simulink subsystem "StreetLaneSegment1x2_asSubsystem"  (R2021a)
settings: Solver=VariableStepAuto  StartTime=0.0  StopTime=10.0  RelTol=1e-3
settings Model: Creator=phill  LastModifiedBy=phill

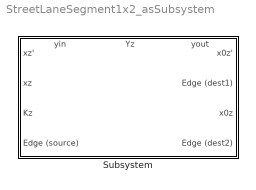
== system StreetLaneSegment1x2_asSubsystem ==
  Subsystem : Subsystem  mask{Kz=0, Tz=0}
      mask prompts: Kz "Kz (Capacity - How many cars fit into this cell)"; Tz "Tz (Nominal travel time for vehicles traveling unobstructed through the cell)"
      mask help: 1x2 Version of the 1x1 default cell.
      settings: PortSchema="{\"entries\":[{\"content\":{\"sides\":[{\"content\":{\"connectorIds\":[\"Out6\",\"Out7\",\"Out8\",\"In1\"]},\"type\":\"ConnectorPlacement.EquallySpacedRectSide\",\"uuid\":\"c6485919-43c0-4a3b-9a67-3a50a1748552\"},{\"content\":{\"connectorIds\":[\"Out1\",\"In2\",\"Out2\",\"In3\"],\"side\":\"RIGHT\"},\"type\":\"ConnectorPlacement.EquallySpacedRectSide\",\"uuid\":\"e12fc750-a76b-4a52-a085-56205ebef983\"},{\"content\":{\"connectorIds\":[\"Out3\",\"Out4\",\"Out5\"],\"side\":\"TOP\"},\"type\":\"ConnectorPlacement.EquallySpacedRectSide\",\"uuid\":\"04ec9430-4292-4c0e-9b60-ad78ee5b6ee3\"}]},\"type\":\"ConnectorPlacement.EquallySpacedConnector\",\"uuid\":\"8d657383-4de4-4f3e-906b-2968264a5f3c\"}],\"packageUris\":[\"http://schema.mathworks.com/mf0/Connector/R2020b\"],\"version\":\"1.0\"}"
      mask Display:
      | image('$imagefile'); % Use "Edit Image" on toolstrip to change.
      | %image('.\LaneIconLightGrey.png');
      | disp('Street Lane Segment 1x2 \n\n');
      | disp(['Kz = ', get_param(gcb,'Kz'), ' | Tz = ', get_param(gcb, 'Tz')])

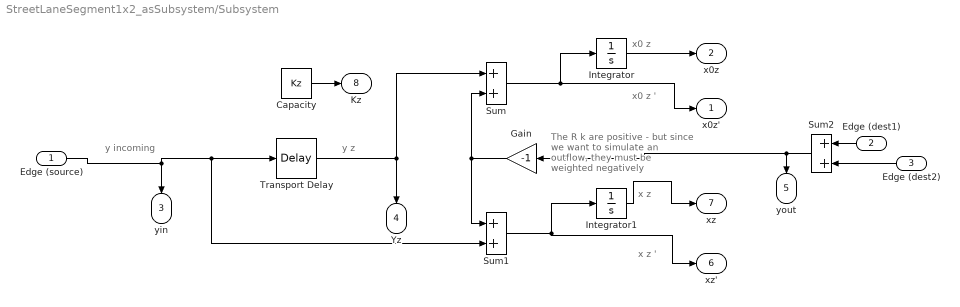
== system StreetLaneSegment1x2_asSubsystem/Subsystem ==
  note: The R k are positive - but since we
      | want to simulate an outflow, they
      | must be weighted negatively
  note: x0 z '
  note: y incoming
  note: y z
  note: x z
  note: x0 z
  note: x z '
  Edge (source) : Inport
  Edge (dest1) : Inport  Port=2
  Edge (dest2) : Inport  Port=3
  Capacity : Constant  Value=Kz
  Gain : Gain  Gain=-1
  Integrator : Integrator
  Integrator1 : Integrator
  Sum : Sum
  Sum1 : Sum
  Sum2 : Sum
  Transport Delay : TransportDelay  DelayTime=Tz
  x0z' : Outport
  x0z : Outport  Port=2
  yin : Outport  Port=3
  Yz : Outport  Port=4
  yout : Outport  Port=5
  xz' : Outport  Port=6
  xz : Outport  Port=7
  Kz : Outport  Port=8
  wires:
  Edge (source)/1 -> yin/1, Sum1/2, Transport Delay/1
  Sum1/1 -> xz'/1, Integrator1/1
  Integrator/1 -> x0z/1
  Transport Delay/1 -> Yz/1, Sum/1
  Capacity/1 -> Kz/1
  Sum2/1 -> Gain/1, yout/1
  Integrator1/1 -> xz/1
  Edge (dest1)/1 -> Sum2/1
  Sum/1 -> x0z'/1, Integrator/1
  Edge (dest2)/1 -> Sum2/2
  Gain/1 -> Sum1/1, Sum/2
